simulink model "Model2"  (R2018b)
settings: Solver=VariableStepAuto  StartTime=0.0  StopTime=30  RelTol=1e-3
undefined symbols (not defined in the file or in its folder): motormaxtorque, motorspeedradps
libraries: simulink x1
settings Model: Creator=sm6814  LastModifiedBy=v12st
settings DebuggingCC: LibraryContextMissingDiagnostic=none
settings SFSimCC: SimUseLocalCustomCode=off
settings RTWCC: RTWUseLocalCustomCode=off

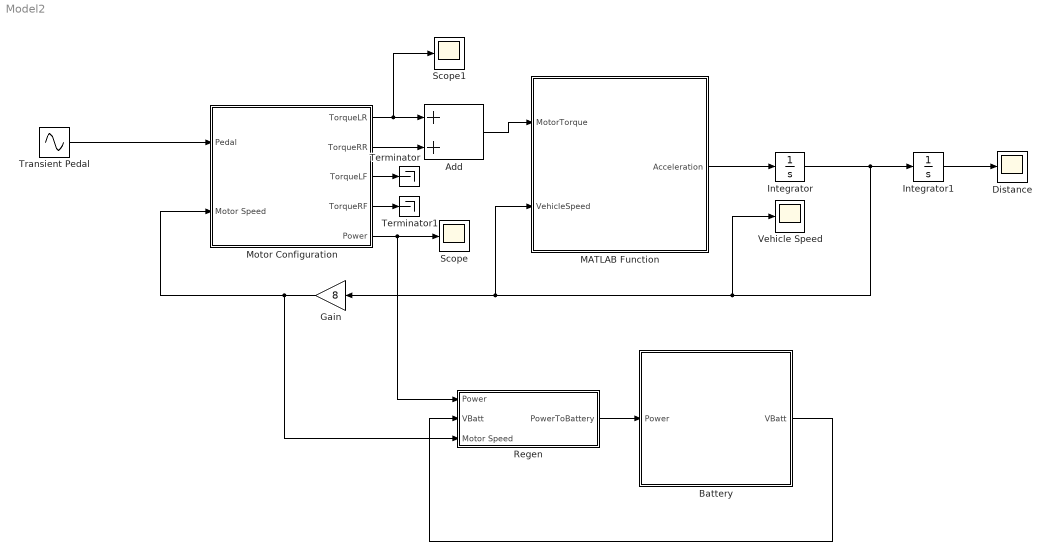
== system Model2 ==
  Add : Sum
  Battery : Subsystem
  "Distance " : Scope
  Gain : Gain  Gain=8
  Integrator : Integrator
  Integrator1 : Integrator
  MATLAB Function : MATLAB Function  TreatAsAtomicUnit=on
  Motor Configuration : Subsystem  Variant=on
  Regen : Subsystem
  Scope : Scope
  Scope1 : Scope
  Terminator : Terminator
  Terminator1 : Terminator
  Transient Pedal : Sin  Frequency=0.8  SampleTime=0
  Vehicle Speed : Scope
  wires:
  MATLAB Function/1(Acceleration) -> Integrator/1
  Integrator1/1 -> "Distance "/1
  Integrator/1 -> Integrator1/1, Vehicle Speed/1, MATLAB Function/2(VehicleSpeed), Gain/1
  Motor Configuration/2(TorqueRR) -> Add/2
  Motor Configuration/1(TorqueLR) -> Scope1/1, Add/1
  Add/1 -> MATLAB Function/1(MotorTorque)
  Motor Configuration/3(TorqueLF) -> Terminator/1
  Motor Configuration/4(TorqueRF) -> Terminator1/1
  Gain/1 -> Regen/3(Motor Speed), Motor Configuration/2(Motor Speed)
  Motor Configuration/5(Power) -> Regen/1(Power), Scope/1
  Regen/1(PowerToBattery) -> Battery/1(Power)
  Battery/1(VBatt) -> Regen/2(VBatt)
  Transient Pedal/1 -> Motor Configuration/1(Pedal)

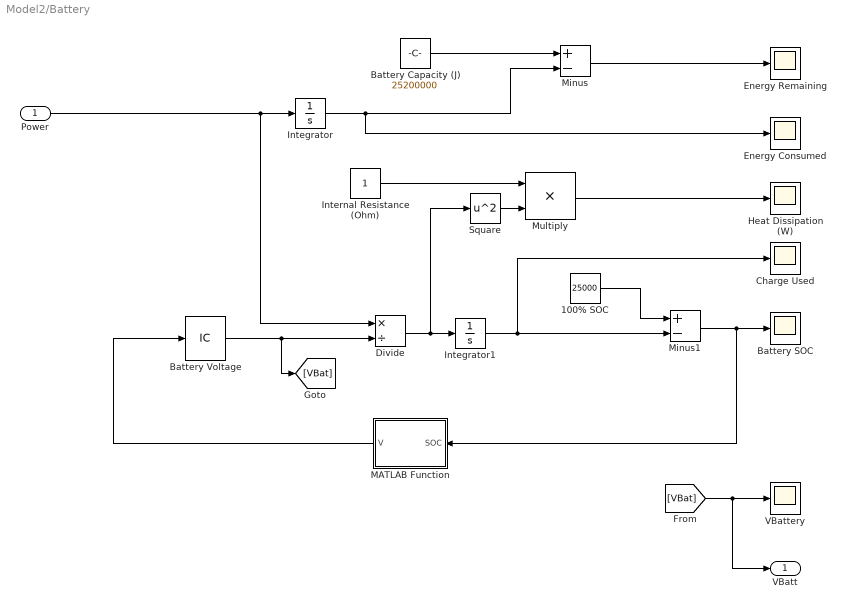
== system Model2/Battery ==
  Power : Inport
  100% SOC : Constant  Value=25000
  Battery Capacity (J) : Constant  Value=25200000
  Battery SOC : Scope
  Battery Voltage : InitialCondition  Value=350
  Charge Used : Scope
  Divide : Product  Inputs=*/
  Energy Consumed : Scope
  Energy Remaining : Scope
  Heat Dissipation (W) : Scope
  Integrator : Integrator
  Integrator1 : Integrator
  Internal Resistance (Ohm) : Constant
  MATLAB Function : MATLAB Function  TreatAsAtomicUnit=on
  Minus : Sum  Inputs=+-
  Minus1 : Sum  Inputs=+-
  Multiply : Product
  Square : Math  Operator=square  SaturateOnIntegerOverflow=on
  VBattery : Scope
  VBatt : Outport
  wires:
  Power/1 -> Divide/1, Integrator/1
  Integrator/1 -> Minus/2, Energy Consumed/1
  Divide/1 -> Square/1, Integrator1/1
  Integrator1/1 -> Charge Used/1, Minus1/2
  Battery Voltage/1 -> [VBat], Divide/2
  Battery Capacity (J)/1 -> Minus/1
  Minus/1 -> Energy Remaining/1
  100% SOC/1 -> Minus1/1
  Minus1/1 -> Battery SOC/1, MATLAB Function/1(SOC)
  MATLAB Function/1(V) -> Battery Voltage/1
  Internal Resistance (Ohm)/1 -> Multiply/1
  Square/1 -> Multiply/2
  Multiply/1 -> Heat Dissipation (W)/1
  [VBat] -> VBatt/1, VBattery/1

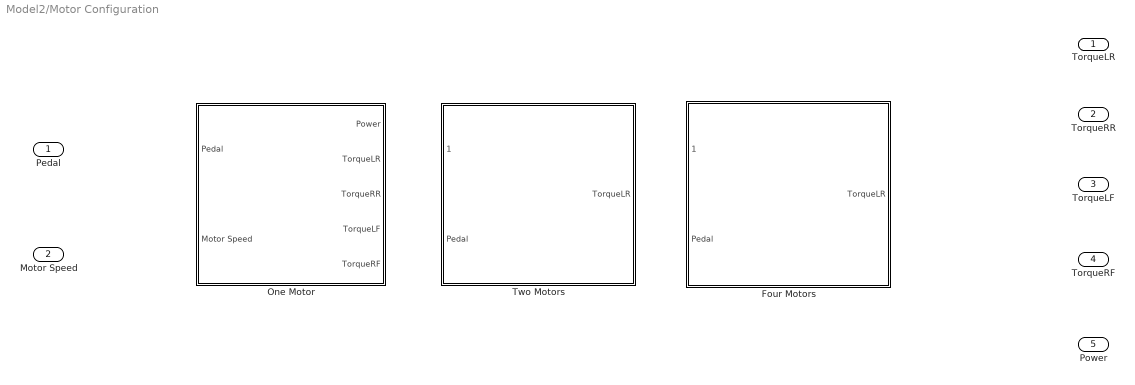
== system Model2/Motor Configuration ==
  Pedal : Inport
  Motor Speed : Inport  Port=2
  Four Motors : Subsystem  VariantControl=FourMotor
  One Motor : Subsystem  VariantControl=OneMotor
  Two Motors : Subsystem  VariantControl=TwoMotor
  TorqueLR : Outport
  TorqueRR : Outport  Port=2
  TorqueLF : Outport  Port=3
  TorqueRF : Outport  Port=4
  Power : Outport  Port=5

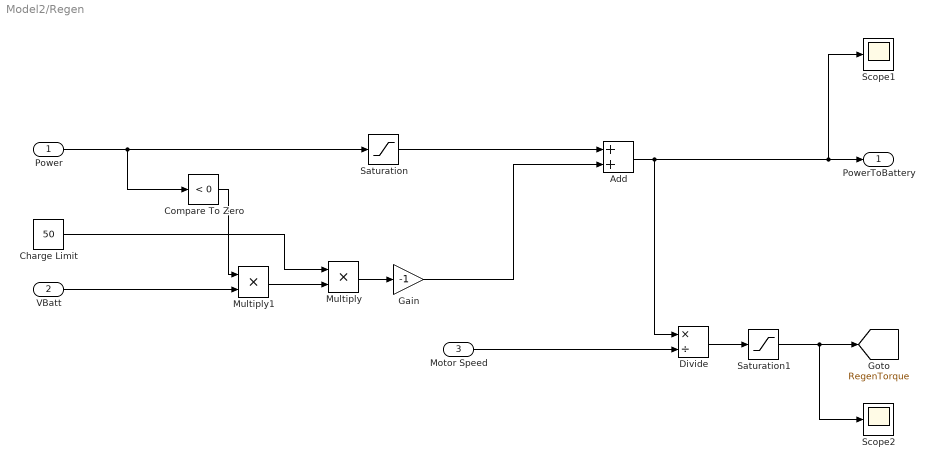
== system Model2/Regen ==
  Power : Inport
  VBatt : Inport  Port=2
  Motor Speed : Inport  Port=3
  Add : Sum
  Charge Limit : Constant  Value=50
  Compare To Zero : simulink/Logic and Bit Operations/Compare To Zero  relop=<  OutDataTypeStr=boolean
  Divide : Product  Inputs=*/
  Gain : Gain  Gain=-1
  Multiply : Product
  Multiply1 : Product
  Saturation : Saturate  UpperLimit=100000  LowerLimit=0
  Saturation1 : Saturate  UpperLimit=0  LowerLimit=-10000
  Scope1 : Scope
  Scope2 : Scope
  PowerToBattery : Outport
  tag scope: RegenTorque=global
  wires:
  Power/1 -> Compare To Zero/1, Saturation/1
  Charge Limit/1 -> Multiply/1
  Saturation/1 -> Add/1
  Add/1 -> Divide/1, Scope1/1, PowerToBattery/1
  VBatt/1 -> Multiply1/2
  Compare To Zero/1 -> Multiply1/1
  Multiply1/1 -> Multiply/2
  Multiply/1 -> Gain/1
  Motor Speed/1 -> Divide/2
  Divide/1 -> Saturation1/1
  Saturation1/1 -> [RegenTorque], Scope2/1
  Gain/1 -> Add/2

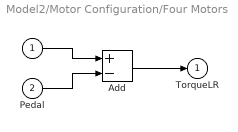
== system Model2/Motor Configuration/Four Motors ==
  " " : Inport
  Pedal : Inport  Port=2
  Add : Sum  Inputs=+-
  TorqueLR : Outport
  wires:
  Pedal/1 -> Add/2
  " "/1 -> Add/1
  Add/1 -> TorqueLR/1

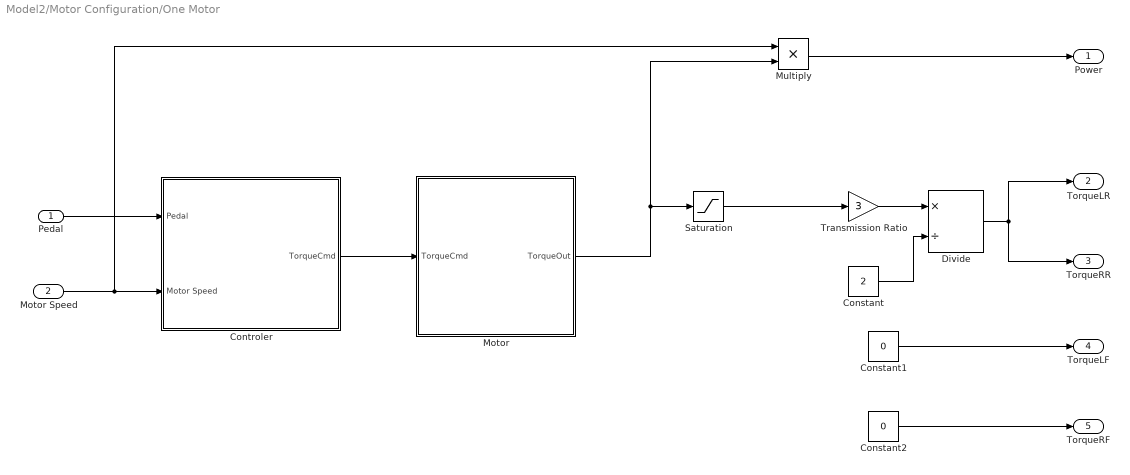
== system Model2/Motor Configuration/One Motor ==
  Pedal : Inport
  Motor Speed : Inport  Port=2
  Constant : Constant  Value=2
  Constant1 : Constant  Value=0
  Constant2 : Constant  Value=0
  Controler : Subsystem
  Divide : Product  Inputs=*/
  Motor : Subsystem
  Multiply : Product
  Saturation : Saturate  UpperLimit=100000  LowerLimit=0
  Transmission Ratio : Gain  Gain=3
  Power : Outport
  TorqueLR : Outport  Port=2
  TorqueRR : Outport  Port=3
  TorqueLF : Outport  Port=4
  TorqueRF : Outport  Port=5
  wires:
  Motor/1(TorqueOut) -> Saturation/1, Multiply/2
  Multiply/1 -> Power/1
  Constant/1 -> Divide/2
  Divide/1 -> TorqueRR/1, TorqueLR/1
  Constant1/1 -> TorqueLF/1
  Constant2/1 -> TorqueRF/1
  Transmission Ratio/1 -> Divide/1
  Pedal/1 -> Controler/1(Pedal)
  Motor Speed/1 -> Controler/2(Motor Speed), Multiply/1
  Controler/1("TorqueCmd ") -> Motor/1(TorqueCmd)
  Saturation/1 -> Transmission Ratio/1

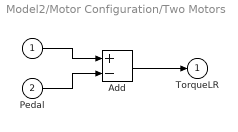
== system Model2/Motor Configuration/Two Motors ==
  " " : Inport
  Pedal : Inport  Port=2
  Add : Sum  Inputs=+-
  TorqueLR : Outport
  wires:
  Pedal/1 -> Add/2
  " "/1 -> Add/1
  Add/1 -> TorqueLR/1

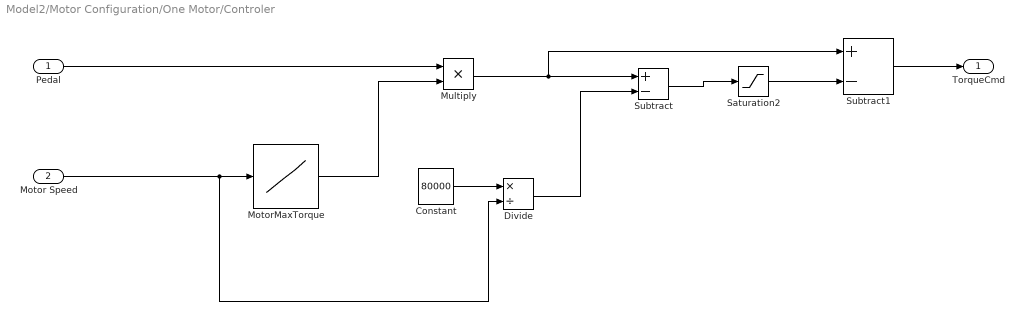
== system Model2/Motor Configuration/One Motor/Controler ==
  Pedal : Inport
  Motor Speed : Inport  Port=2
  Constant : Constant  Value=80000
  Divide : Product  Inputs=*/
  MotorMaxTorque : Lookup_n-D  NumberOfTableDimensions=1  BreakpointsForDimension1=motorspeedradps  Table=motormaxtorque  ExtrapMethod=Clip  InternalRulePriority=Speed  RndMeth=Simplest  InputSameDT=on
  Multiply : Product
  Saturation2 : Saturate  UpperLimit=10000  LowerLimit=0
  Subtract : Sum  Inputs=+-
  Subtract1 : Sum  Inputs=+-
  "TorqueCmd " : Outport
  wires:
  MotorMaxTorque/1 -> Multiply/2
  Pedal/1 -> Multiply/1
  Multiply/1 -> Subtract1/1, Subtract/1
  Divide/1 -> Subtract/2
  Subtract/1 -> Saturation2/1
  Saturation2/1 -> Subtract1/2
  Subtract1/1 -> "TorqueCmd "/1
  Motor Speed/1 -> Divide/2, MotorMaxTorque/1
  Constant/1 -> Divide/1

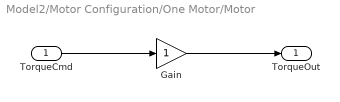
== system Model2/Motor Configuration/One Motor/Motor ==
  TorqueCmd : Inport
  Gain : Gain
  TorqueOut : Outport
  wires:
  TorqueCmd/1 -> Gain/1
  Gain/1 -> TorqueOut/1

== matlab function Model2/Battery/MATLAB Function ==
  data: SOC input; V output
function V = SOCtoVoltage(SOC)

V = 350*(SOC/25000);

== matlab function Model2/MATLAB Function ==
  data: MotorTorque input; Acceleration output; VehicleSpeed input
function Acceleration = Chassis( MotorTorque,VehicleSpeed)

Acceleration=((MotorTorque/(0.2)-0.2*VehicleSpeed^2)/200);
